simulink model "separator"  (R2018b)
settings: Solver=VariableStepAuto  StartTime=0.0  StopTime=100.0  RelTol=1e-3
settings Model: Creator=smf52  LastModifiedBy=art58

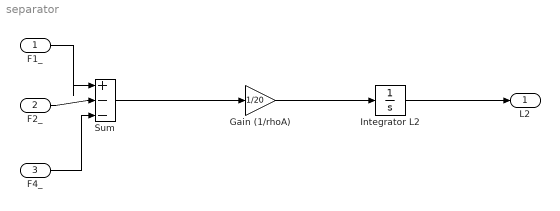
== system separator ==
  F1_ : Inport
  F2_ : Inport  Port=2
  F4_ : Inport  Port=3
  Gain (1/rhoA) : Gain  Gain=1/20
  "Integrator L2 " : Integrator
  Sum : Sum  Inputs=|+--
  "L2 " : Outport
  wires:
  Sum/1 -> Gain (1/rhoA)/1
  Gain (1/rhoA)/1 -> "Integrator L2 "/1
  "Integrator L2 "/1 -> "L2 "/1
  F1_/1 -> Sum/1
  F2_/1 -> Sum/2
  F4_/1 -> Sum/3
